simulink library "temp"  (Simulink 5.0)
undefined symbols (not defined in the file or in its folder): A, A1, B, B1, C, C1, D, D1, F, H, matrix, v1_vec, v2_vec, v3_vec, v_vec
libraries: aerolibschedule x46, simulink3 x46, simulink x18
(part 2 of 2)

== system temp/2D Controller Blend/K1 ==
  e = refs - y : Inport
  index_v1 : Inport  Port=2
  u_measured : Inport  Port=3
  v2 : Inport  Port=4
  Breakpoints v2 : simulink/Look-Up Tables/PreLook-Up Index Search  bpData=breakpoints_v2  searchMode=Binary Search  cacheBpFlag=on  outputFlag=off  extrapMode=Clip to Range  rangeErrorMode=None
  Controller indices1 : Subsystem
  Demux1 : Demux  Outputs=2
  K1 : Subsystem
  K2 : aerolibschedule/2D Controller Blend/K1/K1  SimViewingDevice=off  DataTypeOverride=UseLocalSettings  MinMaxOverflowLogging=UseLocalSettings
      settings: Permissions=ReadWrite  RTWFcnNameOpts=Auto  RTWFileNameOpts=Auto
  K3 : aerolibschedule/2D Controller Blend/K1/K1  SimViewingDevice=off  DataTypeOverride=UseLocalSettings  MinMaxOverflowLogging=UseLocalSettings
      settings: Permissions=ReadWrite  RTWFcnNameOpts=Auto  RTWFileNameOpts=Auto
  Sum1 : Sum  Inputs=+++  SaturateOnIntegerOverflow=on  InputSameDT=on
  lambda1 : Product  SaturateOnIntegerOverflow=on  InputSameDT=on
  lambda2 : Product  SaturateOnIntegerOverflow=on  InputSameDT=on
  lambda3 : Product  SaturateOnIntegerOverflow=on  InputSameDT=on
  u_demand : Outport
  wires:
  u_measured/1 -> K2/4, K3/4, K1/4(u_measured)
  e = refs - y/1 -> K2/1, K3/1, K1/1(e = refs - y)
  lambda2/1 -> Sum1/2
  lambda1/1 -> Sum1/1
  lambda3/1 -> Sum1/3
  K1/1(u_demand) -> lambda1/1
  K2/1 -> lambda2/1
  K3/1 -> lambda3/1
  Sum1/1 -> u_demand/1
  index_v1/1 -> K2/2, K3/2, K1/2(index1)
  Breakpoints v2/1 -> Demux1/1
  v2/1 -> Breakpoints v2/1
  Demux1/1 -> Controller indices1/1(index)
  Demux1/2 -> Controller indices1/2(lambda)
  Controller indices1/1(idx_K1) -> K1/3(index2)
  Controller indices1/2(lambda_K1) -> lambda1/2
  Controller indices1/3(idx_K2) -> K2/3
  Controller indices1/4(lambda_K2) -> lambda2/2
  Controller indices1/5(idx_K3) -> K3/3
  Controller indices1/6(lambda_K3) -> lambda3/2

== system temp/2D Observer Form [A(v),B(v),C(v),F(v),H(v)]/[A,B,C,F,H] ==
  y-y_dem : Inport
  AoA : Inport  Port=2  PortDimensions=2
  Mach : Inport  Port=3  PortDimensions=2
  u_meas : Inport  Port=4
  *A : Product  Multiplication=Matrix(*)  SaturateOnIntegerOverflow=on  InputSameDT=on
  *B : Product  Multiplication=Matrix(*)  SaturateOnIntegerOverflow=on  InputSameDT=on
  *C : Product  Multiplication=Matrix(*)  SaturateOnIntegerOverflow=on  InputSameDT=on
  *F : Product  Orientation=left  Multiplication=Matrix(*)  SaturateOnIntegerOverflow=on  InputSameDT=on
  *H : Product  Orientation=down  Multiplication=Matrix(*)  SaturateOnIntegerOverflow=on  InputSameDT=on
  A : aerolibschedule/Interpolate Matrix(x,y)  matrix=A
  B : aerolibschedule/Interpolate Matrix(x,y)  matrix=B
  C : aerolibschedule/Interpolate Matrix(x,y)  matrix=C
  F : aerolibschedule/Interpolate Matrix(x,y)  matrix=F
  H : aerolibschedule/Interpolate Matrix(x,y)  matrix=H
  Sum : Sum  Orientation=left  Inputs=+|+  SaturateOnIntegerOverflow=on  InputSameDT=on
  Sum1 : Sum  Orientation=down  Inputs=++|  SaturateOnIntegerOverflow=on  InputSameDT=on
  Sum2 : Sum  Orientation=down  Inputs=|++  SaturateOnIntegerOverflow=on  InputSameDT=on
  estimated state : Integrator  Orientation=left  InitialCondition=x_initial
  u_dem : Outport  Orientation=left
  wires:
  u_meas/1 -> *B/2
  Sum/1 -> estimated state/1
  estimated state/1 -> *F/2, *A/2, *C/2
  *A/1 -> Sum/2
  *F/1 -> u_dem/1
  *B/1 -> Sum1/1
  Sum1/1 -> Sum/1
  *H/1 -> Sum1/2
  Sum2/1 -> *H/2
  *C/1 -> Sum2/2
  A/1 -> *A/1
  C/1 -> *C/1
  F/1 -> *F/1
  B/1 -> *B/1
  H/1 -> *H/1
  y-y_dem/1 -> Sum2/1
  AoA/1 -> A/1, C/1, F/1, B/1, H/1
  Mach/1 -> A/2, C/2, F/2, B/2, H/2

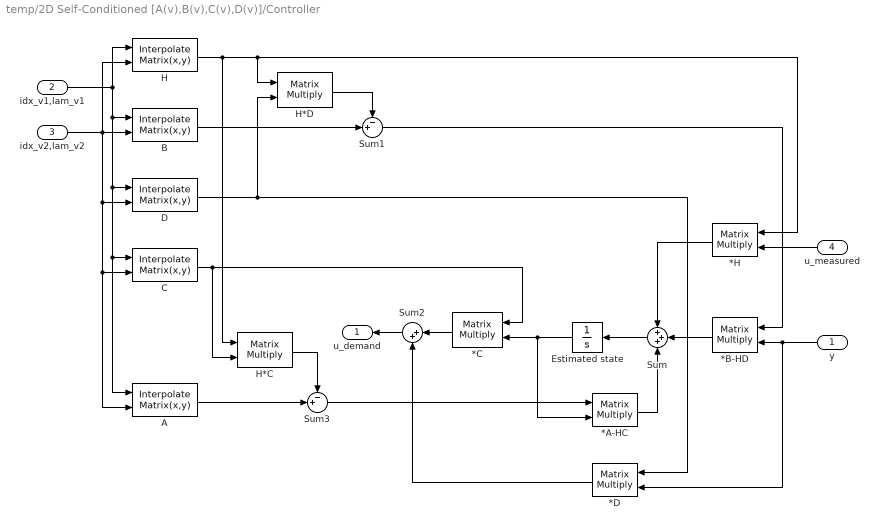
== system temp/2D Self-Conditioned [A(v),B(v),C(v),D(v)]/Controller ==
  y : Inport  Orientation=left
  idx_v1,lam_v1 : Inport  Port=2  PortDimensions=2
  idx_v2,lam_v2 : Inport  Port=3  PortDimensions=2
  u_measured : Inport  Orientation=left  Port=4
  *A-HC : Product  Multiplication=Matrix(*)  SaturateOnIntegerOverflow=on  InputSameDT=on
  *B-HD : Product  Orientation=left  Multiplication=Matrix(*)  SaturateOnIntegerOverflow=on  InputSameDT=on
  *C : Product  Orientation=left  Multiplication=Matrix(*)  SaturateOnIntegerOverflow=on  InputSameDT=on
  *D : Product  Orientation=left  Multiplication=Matrix(*)  SaturateOnIntegerOverflow=on  InputSameDT=on
  *H : Product  Orientation=left  Multiplication=Matrix(*)  SaturateOnIntegerOverflow=on  InputSameDT=on
  A : aerolibschedule/Interpolate Matrix(x,y)  matrix=A
  B : aerolibschedule/Interpolate Matrix(x,y)  matrix=B
  C : aerolibschedule/Interpolate Matrix(x,y)  matrix=C
  D : aerolibschedule/Interpolate Matrix(x,y)  matrix=D
  Estimated state : Integrator  Orientation=left  InitialCondition=x_initial
  H : aerolibschedule/Interpolate Matrix(x,y)  matrix=H
  H*C : Product  Multiplication=Matrix(*)  SaturateOnIntegerOverflow=on  InputSameDT=on
  H*D : Product  Multiplication=Matrix(*)  SaturateOnIntegerOverflow=on  InputSameDT=on
  Sum : Sum  Orientation=left  Inputs=+++  SaturateOnIntegerOverflow=on  InputSameDT=on
  Sum1 : Sum  Inputs=-+|  SaturateOnIntegerOverflow=on  InputSameDT=on
  Sum2 : Sum  Orientation=left  Inputs=|++  SaturateOnIntegerOverflow=on  InputSameDT=on
  Sum3 : Sum  Inputs=-+|  SaturateOnIntegerOverflow=on  InputSameDT=on
  u_demand : Outport  Orientation=left
  wires:
  idx_v2,lam_v2/1 -> C/2, A/2, D/2, H/2, B/2
  H*C/1 -> Sum3/1
  Sum3/1 -> *A-HC/1
  A/1 -> Sum3/2
  Sum1/1 -> *B-HD/1
  B/1 -> Sum1/2
  H*D/1 -> Sum1/1
  H/1 -> H*C/1, H*D/1, *H/1
  u_measured/1 -> *H/2
  *H/1 -> Sum/1
  *B-HD/1 -> Sum/2
  *A-HC/1 -> Sum/3
  Sum/1 -> Estimated state/1
  Estimated state/1 -> *C/2, *A-HC/2
  C/1 -> H*C/2, *C/1
  y/1 -> *B-HD/2, *D/2
  idx_v1,lam_v1/1 -> H/1, B/1, C/1, A/1, D/1
  *C/1 -> Sum2/1
  *D/1 -> Sum2/2
  Sum2/1 -> u_demand/1
  D/1 -> H*D/2, *D/1

== system temp/3D Controller [A(v),B(v),C(v),D(v)]/[A,B,C,D] ==
  y : Inport  Orientation=left
  AoA : Inport  Port=2  PortDimensions=2
  AoS : Inport  Port=3  PortDimensions=2
  Mach : Inport  Port=4  PortDimensions=2
  *A : Product  Multiplication=Matrix(*)  SaturateOnIntegerOverflow=on  InputSameDT=on
  *B : Product  Orientation=left  Multiplication=Matrix(*)  SaturateOnIntegerOverflow=on  InputSameDT=on
  *C : Product  Orientation=left  Multiplication=Matrix(*)  SaturateOnIntegerOverflow=on  InputSameDT=on
  *D : Product  Orientation=left  Multiplication=Matrix(*)  SaturateOnIntegerOverflow=on  InputSameDT=on
  A : aerolibschedule/Interpolate Matrix(x,y,z)  matrix=A
  B : aerolibschedule/Interpolate Matrix(x,y,z)  matrix=B
  C : aerolibschedule/Interpolate Matrix(x,y,z)  matrix=C
  D : aerolibschedule/Interpolate Matrix(x,y,z)  matrix=D
  Estimated state : Integrator  Orientation=left  InitialCondition=x_initial
  Sum : Sum  Orientation=left  Inputs=|++  SaturateOnIntegerOverflow=on  InputSameDT=on
  Sum2 : Sum  Orientation=left  Inputs=|++  SaturateOnIntegerOverflow=on  InputSameDT=on
  u : Outport  Orientation=left
  wires:
  D/1 -> *D/1
  Sum2/1 -> u/1
  *D/1 -> Sum2/2
  *C/1 -> Sum2/1
  Mach/1 -> C/3, A/3, D/3, B/3
  AoS/1 -> C/2, A/2, D/2, B/2
  AoA/1 -> C/1, A/1, D/1, B/1
  y/1 -> *D/2, *B/2
  B/1 -> *B/1
  C/1 -> *C/1
  A/1 -> *A/1
  *B/1 -> Sum/1
  *A/1 -> Sum/2
  Estimated state/1 -> *A/2, *C/2
  Sum/1 -> Estimated state/1

== system temp/3D Observer Form [A(v),B(v),C(v),F(v),H(v)]/[A,B,C,F,H] ==
  y-y_dem : Inport
  AoA : Inport  Port=2  PortDimensions=2
  AoS : Inport  Port=3  PortDimensions=2
  Mach : Inport  Port=4  PortDimensions=2
  u_meas : Inport  Port=5
  *A : Product  Multiplication=Matrix(*)  SaturateOnIntegerOverflow=on  InputSameDT=on
  *B : Product  Multiplication=Matrix(*)  SaturateOnIntegerOverflow=on  InputSameDT=on
  *C : Product  Multiplication=Matrix(*)  SaturateOnIntegerOverflow=on  InputSameDT=on
  *F : Product  Orientation=left  Multiplication=Matrix(*)  SaturateOnIntegerOverflow=on  InputSameDT=on
  *H : Product  Orientation=down  Multiplication=Matrix(*)  SaturateOnIntegerOverflow=on  InputSameDT=on
  A : aerolibschedule/Interpolate Matrix(x,y,z)  matrix=A
  B : aerolibschedule/Interpolate Matrix(x,y,z)  matrix=B
  C : aerolibschedule/Interpolate Matrix(x,y,z)  matrix=C
  F : aerolibschedule/Interpolate Matrix(x,y,z)  matrix=F
  H : aerolibschedule/Interpolate Matrix(x,y,z)  matrix=H
  Sum : Sum  Orientation=left  Inputs=+|+  SaturateOnIntegerOverflow=on  InputSameDT=on
  Sum1 : Sum  Orientation=down  Inputs=++|  SaturateOnIntegerOverflow=on  InputSameDT=on
  Sum2 : Sum  Orientation=down  Inputs=|++  SaturateOnIntegerOverflow=on  InputSameDT=on
  estimated state : Integrator  Orientation=left  InitialCondition=x_initial
  u_dem : Outport  Orientation=left
  wires:
  u_meas/1 -> *B/2
  Mach/1 -> A/3, C/3, F/3, B/3, H/3
  AoS/1 -> A/2, C/2, F/2, B/2, H/2
  AoA/1 -> A/1, C/1, F/1, B/1, H/1
  y-y_dem/1 -> Sum2/1
  H/1 -> *H/1
  B/1 -> *B/1
  F/1 -> *F/1
  C/1 -> *C/1
  A/1 -> *A/1
  *C/1 -> Sum2/2
  Sum2/1 -> *H/2
  *H/1 -> Sum1/2
  Sum1/1 -> Sum/1
  *B/1 -> Sum1/1
  *F/1 -> u_dem/1
  *A/1 -> Sum/2
  estimated state/1 -> *C/2, *A/2, *F/2
  Sum/1 -> estimated state/1

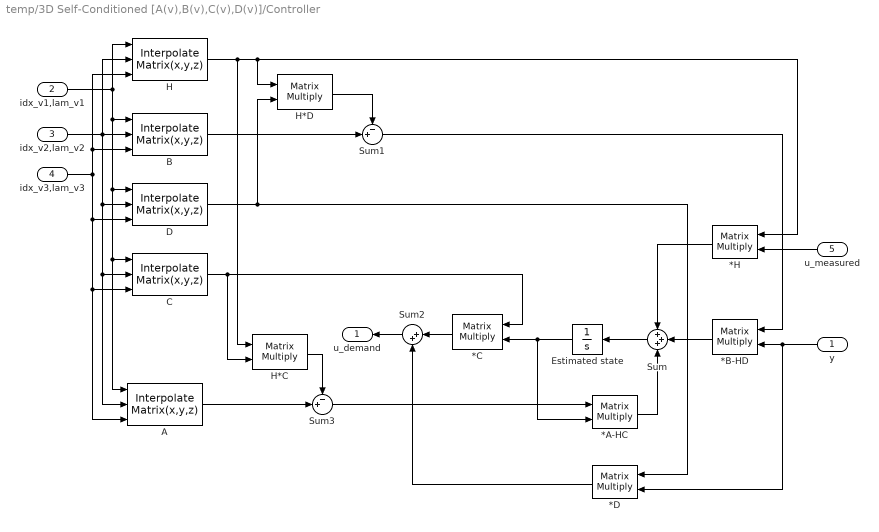
== system temp/3D Self-Conditioned [A(v),B(v),C(v),D(v)]/Controller ==
  y : Inport  Orientation=left
  idx_v1,lam_v1 : Inport  Port=2  PortDimensions=2
  idx_v2,lam_v2 : Inport  Port=3  PortDimensions=2
  idx_v3,lam_v3 : Inport  Port=4  PortDimensions=2
  u_measured : Inport  Orientation=left  Port=5
  *A-HC : Product  Multiplication=Matrix(*)  SaturateOnIntegerOverflow=on  InputSameDT=on
  *B-HD : Product  Orientation=left  Multiplication=Matrix(*)  SaturateOnIntegerOverflow=on  InputSameDT=on
  *C : Product  Orientation=left  Multiplication=Matrix(*)  SaturateOnIntegerOverflow=on  InputSameDT=on
  *D : Product  Orientation=left  Multiplication=Matrix(*)  SaturateOnIntegerOverflow=on  InputSameDT=on
  *H : Product  Orientation=left  Multiplication=Matrix(*)  SaturateOnIntegerOverflow=on  InputSameDT=on
  A : aerolibschedule/Interpolate Matrix(x,y,z)  matrix=A
  B : aerolibschedule/Interpolate Matrix(x,y,z)  matrix=B
  C : aerolibschedule/Interpolate Matrix(x,y,z)  matrix=C
  D : aerolibschedule/Interpolate Matrix(x,y,z)  matrix=D
  Estimated state : Integrator  Orientation=left  InitialCondition=x_initial
  H : aerolibschedule/Interpolate Matrix(x,y,z)  matrix=H
  H*C : Product  Multiplication=Matrix(*)  SaturateOnIntegerOverflow=on  InputSameDT=on
  H*D : Product  Multiplication=Matrix(*)  SaturateOnIntegerOverflow=on  InputSameDT=on
  Sum : Sum  Orientation=left  Inputs=+++  SaturateOnIntegerOverflow=on  InputSameDT=on
  Sum1 : Sum  Inputs=-+|  SaturateOnIntegerOverflow=on  InputSameDT=on
  Sum2 : Sum  Orientation=left  Inputs=|++  SaturateOnIntegerOverflow=on  InputSameDT=on
  Sum3 : Sum  Inputs=-+|  SaturateOnIntegerOverflow=on  InputSameDT=on
  u_demand : Outport  Orientation=left
  wires:
  idx_v3,lam_v3/1 -> C/3, A/3, D/3, H/3, B/3
  D/1 -> *D/1, H*D/2
  Sum2/1 -> u_demand/1
  *D/1 -> Sum2/2
  *C/1 -> Sum2/1
  idx_v1,lam_v1/1 -> C/1, A/1, D/1, H/1, B/1
  y/1 -> *D/2, *B-HD/2
  C/1 -> *C/1, H*C/2
  Estimated state/1 -> *A-HC/2, *C/2
  Sum/1 -> Estimated state/1
  *A-HC/1 -> Sum/3
  *B-HD/1 -> Sum/2
  *H/1 -> Sum/1
  u_measured/1 -> *H/2
  H/1 -> *H/1, H*D/1, H*C/1
  H*D/1 -> Sum1/1
  B/1 -> Sum1/2
  Sum1/1 -> *B-HD/1
  A/1 -> Sum3/2
  Sum3/1 -> *A-HC/1
  H*C/1 -> Sum3/1
  idx_v2,lam_v2/1 -> C/2, A/2, D/2, H/2, B/2

== system temp/Interpolate Matrix(x)/Matrix interpolation ==
  index : Inport
  lambda_x : Inport  Orientation=down  Port=2  PortDimensions=1
  1-lambda_x : Product  SaturateOnIntegerOverflow=on  InputSameDT=on
  Fcn : Fcn  Expr=1-u(1)
  Sum : Sum  Inputs=|++  SaturateOnIntegerOverflow=on  InputSameDT=on
  Sum3 : Sum  Inputs=+|+  SaturateOnIntegerOverflow=on  InputSameDT=on
  "[0]" : simulink3/Functions & Tables/Direct Look-Up Table (n-D)  maskTabDims=More...  explicitNumDims=3  outDims=2-D Matrix  tabIsInput=off  mxTable=matrix  clipFlag=Warning
  "[1]" : simulink3/Functions & Tables/Direct Look-Up Table (n-D)  maskTabDims=More...  explicitNumDims=3  outDims=2-D Matrix  tabIsInput=off  mxTable=matrix  clipFlag=Warning
  lambda_x. : Product  SaturateOnIntegerOverflow=on  InputSameDT=on
  offset for upper index 1 : Constant
  matrix : Outport
  wires:
  Sum3/1 -> matrix/1
  lambda_x./1 -> Sum3/2
  1-lambda_x/1 -> Sum3/1
  Fcn/1 -> 1-lambda_x/2
  "[1]"/1 -> lambda_x./1
  "[0]"/1 -> 1-lambda_x/1
  Sum/1 -> "[1]"/1
  offset for upper index 1/1 -> Sum/2
  index/1 -> "[0]"/1, Sum/1
  lambda_x/1 -> lambda_x./2, Fcn/1

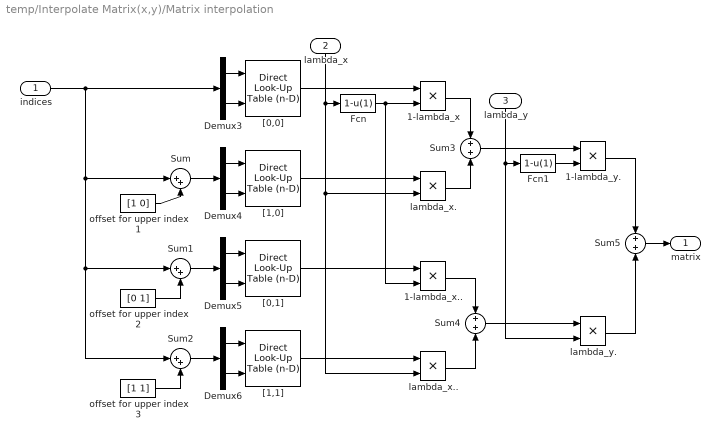
== system temp/Interpolate Matrix(x,y)/Matrix interpolation ==
  indices : Inport
  lambda_x : Inport  Orientation=down  Port=2
  lambda_y : Inport  Orientation=down  Port=3
  1-lambda_x : Product  SaturateOnIntegerOverflow=on  InputSameDT=on
  1-lambda_x.. : Product  SaturateOnIntegerOverflow=on  InputSameDT=on
  1-lambda_y. : Product  SaturateOnIntegerOverflow=on  InputSameDT=on
  Demux{3..6} (4 alike) : Demux  Outputs=2
  Fcn : Fcn  Expr=1-u(1)
  Fcn1 : Fcn  Expr=1-u(1)
  Sum : Sum  Inputs=|++  SaturateOnIntegerOverflow=on  InputSameDT=on
  Sum1 : Sum  Inputs=|++  SaturateOnIntegerOverflow=on  InputSameDT=on
  Sum2 : Sum  Inputs=|++  SaturateOnIntegerOverflow=on  InputSameDT=on
  Sum3 : Sum  Inputs=+|+  SaturateOnIntegerOverflow=on  InputSameDT=on
  Sum4 : Sum  Inputs=+|+  SaturateOnIntegerOverflow=on  InputSameDT=on
  Sum5 : Sum  Inputs=+|+  SaturateOnIntegerOverflow=on  InputSameDT=on
  "[0,0]" : simulink3/Functions & Tables/Direct Look-Up Table (n-D)  maskTabDims=More...  explicitNumDims=4  outDims=2-D Matrix  tabIsInput=off  mxTable=matrix  clipFlag=Warning
  "[0,1]" : simulink3/Functions & Tables/Direct Look-Up Table (n-D)  maskTabDims=More...  explicitNumDims=4  outDims=2-D Matrix  tabIsInput=off  mxTable=matrix  clipFlag=Warning
  "[1,0]" : simulink3/Functions & Tables/Direct Look-Up Table (n-D)  maskTabDims=More...  explicitNumDims=4  outDims=2-D Matrix  tabIsInput=off  mxTable=matrix  clipFlag=Warning
  "[1,1]" : simulink3/Functions & Tables/Direct Look-Up Table (n-D)  maskTabDims=More...  explicitNumDims=4  outDims=2-D Matrix  tabIsInput=off  mxTable=matrix  clipFlag=Warning
  lambda_x. : Product  SaturateOnIntegerOverflow=on  InputSameDT=on
  lambda_x.. : Product  SaturateOnIntegerOverflow=on  InputSameDT=on
  lambda_y. : Product  SaturateOnIntegerOverflow=on  InputSameDT=on
  offset for upper index 1 : Constant  Value=[1 0]
  offset for upper index 2 : Constant  Value=[0 1]
  offset for upper index 3 : Constant  Value=[1 1]
  matrix : Outport
  wires:
  lambda_x/1 -> lambda_x../2, lambda_x./2, Fcn/1
  lambda_y/1 -> lambda_y./2, Fcn1/1
  Sum5/1 -> matrix/1
  indices/1 -> Sum2/1, Sum1/1, Sum/1, Demux3/1
  offset for upper index 3/1 -> Sum2/2
  Sum2/1 -> Demux6/1
  Demux6/2 -> "[1,1]"/2
  Demux6/1 -> "[1,1]"/1
  offset for upper index 2/1 -> Sum1/2
  Sum1/1 -> Demux5/1
  Demux5/2 -> "[0,1]"/2
  Demux5/1 -> "[0,1]"/1
  offset for upper index 1/1 -> Sum/2
  Sum/1 -> Demux4/1
  Demux4/2 -> "[1,0]"/2
  Demux4/1 -> "[1,0]"/1
  Demux3/2 -> "[0,0]"/2
  Demux3/1 -> "[0,0]"/1
  "[0,0]"/1 -> 1-lambda_x/1
  "[1,0]"/1 -> lambda_x./1
  "[0,1]"/1 -> 1-lambda_x../1
  "[1,1]"/1 -> lambda_x../1
  Fcn/1 -> 1-lambda_x/2, 1-lambda_x../2
  1-lambda_x/1 -> Sum3/1
  lambda_x./1 -> Sum3/2
  1-lambda_x../1 -> Sum4/1
  lambda_x../1 -> Sum4/2
  Sum3/1 -> 1-lambda_y./1
  Sum4/1 -> lambda_y./1
  Fcn1/1 -> 1-lambda_y./2
  1-lambda_y./1 -> Sum5/1
  lambda_y./1 -> Sum5/2

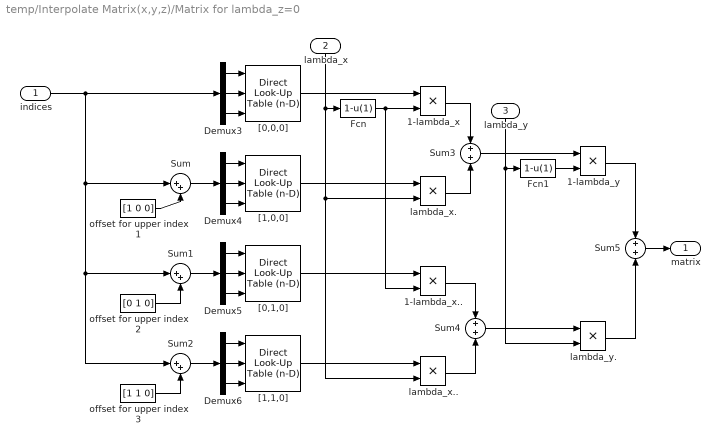
== system temp/Interpolate Matrix(x,y,z)/Matrix for lambda_z=0 ==
  indices : Inport
  lambda_x : Inport  Orientation=down  Port=2
  lambda_y : Inport  Orientation=down  Port=3
  1-lambda_x : Product  SaturateOnIntegerOverflow=on  InputSameDT=on
  1-lambda_x.. : Product  SaturateOnIntegerOverflow=on  InputSameDT=on
  1-lambda_y : Product  SaturateOnIntegerOverflow=on  InputSameDT=on
  Demux{3..6} (4 alike) : Demux  Outputs=3
  Fcn : Fcn  Expr=1-u(1)
  Fcn1 : Fcn  Expr=1-u(1)
  Sum : Sum  Inputs=|++  SaturateOnIntegerOverflow=on  InputSameDT=on
  Sum1 : Sum  Inputs=|++  SaturateOnIntegerOverflow=on  InputSameDT=on
  Sum2 : Sum  Inputs=|++  SaturateOnIntegerOverflow=on  InputSameDT=on
  Sum3 : Sum  Inputs=+|+  SaturateOnIntegerOverflow=on  InputSameDT=on
  Sum4 : Sum  Inputs=+|+  SaturateOnIntegerOverflow=on  InputSameDT=on
  Sum5 : Sum  Inputs=+|+  SaturateOnIntegerOverflow=on  InputSameDT=on
  "[0,0,0]" : simulink3/Functions & Tables/Direct Look-Up Table (n-D)  maskTabDims=More...  explicitNumDims=5  outDims=2-D Matrix  tabIsInput=off  mxTable=matrix  clipFlag=Warning
  "[0,1,0]" : simulink3/Functions & Tables/Direct Look-Up Table (n-D)  maskTabDims=More...  explicitNumDims=5  outDims=2-D Matrix  tabIsInput=off  mxTable=matrix  clipFlag=Warning
  "[1,0,0]" : simulink3/Functions & Tables/Direct Look-Up Table (n-D)  maskTabDims=More...  explicitNumDims=5  outDims=2-D Matrix  tabIsInput=off  mxTable=matrix  clipFlag=Warning
  "[1,1,0]" : simulink3/Functions & Tables/Direct Look-Up Table (n-D)  maskTabDims=More...  explicitNumDims=5  outDims=2-D Matrix  tabIsInput=off  mxTable=matrix  clipFlag=Warning
  lambda_x. : Product  SaturateOnIntegerOverflow=on  InputSameDT=on
  lambda_x.. : Product  SaturateOnIntegerOverflow=on  InputSameDT=on
  lambda_y. : Product  SaturateOnIntegerOverflow=on  InputSameDT=on
  offset for upper index 1 : Constant  Value=[1 0 0]
  offset for upper index 2 : Constant  Value=[0 1 0]
  offset for upper index 3 : Constant  Value=[1 1 0]
  matrix : Outport
  wires:
  lambda_x/1 -> lambda_x../2, lambda_x./2, Fcn/1
  lambda_y/1 -> lambda_y./2, Fcn1/1
  lambda_y./1 -> Sum5/2
  1-lambda_y/1 -> Sum5/1
  Fcn1/1 -> 1-lambda_y/2
  Sum4/1 -> lambda_y./1
  Sum3/1 -> 1-lambda_y/1
  lambda_x../1 -> Sum4/2
  1-lambda_x../1 -> Sum4/1
  lambda_x./1 -> Sum3/2
  1-lambda_x/1 -> Sum3/1
  Fcn/1 -> 1-lambda_x../2, 1-lambda_x/2
  "[1,1,0]"/1 -> lambda_x../1
  "[0,1,0]"/1 -> 1-lambda_x../1
  "[1,0,0]"/1 -> lambda_x./1
  "[0,0,0]"/1 -> 1-lambda_x/1
  Demux3/1 -> "[0,0,0]"/1
  Demux3/2 -> "[0,0,0]"/2
  Demux3/3 -> "[0,0,0]"/3
  Demux4/1 -> "[1,0,0]"/1
  Demux4/2 -> "[1,0,0]"/2
  Sum/1 -> Demux4/1
  Demux4/3 -> "[1,0,0]"/3
  offset for upper index 1/1 -> Sum/2
  Demux5/1 -> "[0,1,0]"/1
  Demux5/2 -> "[0,1,0]"/2
  Demux5/3 -> "[0,1,0]"/3
  Sum1/1 -> Demux5/1
  offset for upper index 2/1 -> Sum1/2
  Demux6/1 -> "[1,1,0]"/1
  Demux6/2 -> "[1,1,0]"/2
  Demux6/3 -> "[1,1,0]"/3
  Sum2/1 -> Demux6/1
  offset for upper index 3/1 -> Sum2/2
  indices/1 -> Demux3/1, Sum/1, Sum1/1, Sum2/1
  Sum5/1 -> matrix/1

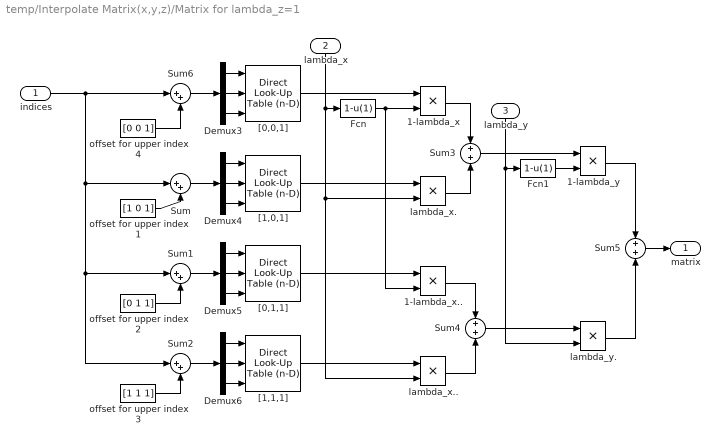
== system temp/Interpolate Matrix(x,y,z)/Matrix for lambda_z=1 ==
  indices : Inport
  lambda_x : Inport  Orientation=down  Port=2
  lambda_y : Inport  Orientation=down  Port=3
  1-lambda_x : Product  SaturateOnIntegerOverflow=on  InputSameDT=on
  1-lambda_x.. : Product  SaturateOnIntegerOverflow=on  InputSameDT=on
  1-lambda_y : Product  SaturateOnIntegerOverflow=on  InputSameDT=on
  Demux{3..6} (4 alike) : Demux  Outputs=3
  Fcn : Fcn  Expr=1-u(1)
  Fcn1 : Fcn  Expr=1-u(1)
  Sum{,1..2,6} (4 alike) : Sum  Inputs=|++  SaturateOnIntegerOverflow=on  InputSameDT=on
  Sum3 : Sum  Inputs=+|+  SaturateOnIntegerOverflow=on  InputSameDT=on
  Sum4 : Sum  Inputs=+|+  SaturateOnIntegerOverflow=on  InputSameDT=on
  Sum5 : Sum  Inputs=+|+  SaturateOnIntegerOverflow=on  InputSameDT=on
  "[0,0,1]" : simulink3/Functions & Tables/Direct Look-Up Table (n-D)  maskTabDims=More...  explicitNumDims=5  outDims=2-D Matrix  tabIsInput=off  mxTable=matrix  clipFlag=Warning
  "[0,1,1]" : simulink3/Functions & Tables/Direct Look-Up Table (n-D)  maskTabDims=More...  explicitNumDims=5  outDims=2-D Matrix  tabIsInput=off  mxTable=matrix  clipFlag=Warning
  "[1,0,1]" : simulink3/Functions & Tables/Direct Look-Up Table (n-D)  maskTabDims=More...  explicitNumDims=5  outDims=2-D Matrix  tabIsInput=off  mxTable=matrix  clipFlag=Warning
  "[1,1,1]" : simulink3/Functions & Tables/Direct Look-Up Table (n-D)  maskTabDims=More...  explicitNumDims=5  outDims=2-D Matrix  tabIsInput=off  mxTable=matrix  clipFlag=Warning
  lambda_x. : Product  SaturateOnIntegerOverflow=on  InputSameDT=on
  lambda_x.. : Product  SaturateOnIntegerOverflow=on  InputSameDT=on
  lambda_y. : Product  SaturateOnIntegerOverflow=on  InputSameDT=on
  offset for upper index 1 : Constant  Value=[1 0 1]
  offset for upper index 2 : Constant  Value=[0 1 1]
  offset for upper index 3 : Constant  Value=[1 1 1]
  offset for upper index 4 : Constant  Value=[0 0 1]
  matrix : Outport
  wires:
  offset for upper index 4/1 -> Sum6/2
  Sum6/1 -> Demux3/1
  Sum5/1 -> matrix/1
  indices/1 -> Sum6/1, Sum2/1, Sum1/1, Sum/1
  offset for upper index 3/1 -> Sum2/2
  Sum2/1 -> Demux6/1
  Demux6/3 -> "[1,1,1]"/3
  Demux6/2 -> "[1,1,1]"/2
  Demux6/1 -> "[1,1,1]"/1
  offset for upper index 2/1 -> Sum1/2
  Sum1/1 -> Demux5/1
  Demux5/3 -> "[0,1,1]"/3
  Demux5/2 -> "[0,1,1]"/2
  Demux5/1 -> "[0,1,1]"/1
  offset for upper index 1/1 -> Sum/2
  Demux4/3 -> "[1,0,1]"/3
  Sum/1 -> Demux4/1
  Demux4/2 -> "[1,0,1]"/2
  Demux4/1 -> "[1,0,1]"/1
  Demux3/3 -> "[0,0,1]"/3
  Demux3/2 -> "[0,0,1]"/2
  Demux3/1 -> "[0,0,1]"/1
  "[0,0,1]"/1 -> 1-lambda_x/1
  "[1,0,1]"/1 -> lambda_x./1
  "[0,1,1]"/1 -> 1-lambda_x../1
  "[1,1,1]"/1 -> lambda_x../1
  Fcn/1 -> 1-lambda_x/2, 1-lambda_x../2
  1-lambda_x/1 -> Sum3/1
  lambda_x./1 -> Sum3/2
  1-lambda_x../1 -> Sum4/1
  lambda_x../1 -> Sum4/2
  Sum3/1 -> 1-lambda_y/1
  Sum4/1 -> lambda_y./1
  Fcn1/1 -> 1-lambda_y/2
  1-lambda_y/1 -> Sum5/1
  lambda_y./1 -> Sum5/2
  lambda_y/1 -> Fcn1/1, lambda_y./2
  lambda_x/1 -> Fcn/1, lambda_x./2, lambda_x../2

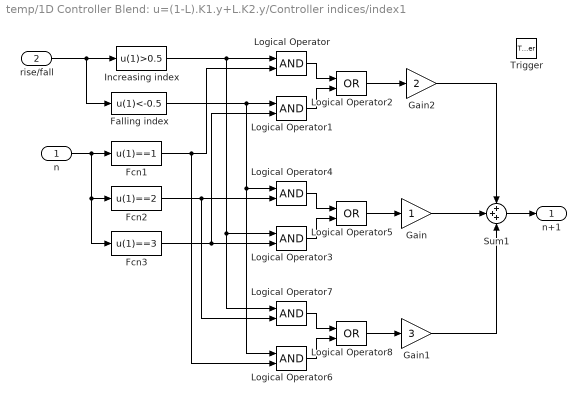
== system temp/1D Controller Blend: u=(1-L).K1.y+L.K2.y/Controller indices/index1 ==
  n : Inport
  rise/fall : Inport  Port=2
  Trigger : TriggerPort
  Falling index : Fcn  Expr=u(1)<-0.5
  Fcn1 : Fcn  Expr=u(1)==1
  Fcn2 : Fcn  Expr=u(1)==2
  Fcn3 : Fcn  Expr=u(1)==3
  Gain : Gain  SaturateOnIntegerOverflow=on
  Gain1 : Gain  Gain=3  SaturateOnIntegerOverflow=on
  Gain2 : Gain  Gain=2  SaturateOnIntegerOverflow=on
  Increasing index : Fcn  Expr=u(1)>0.5
  Logical Operator{,1,3..4,6..7} (6 alike) : Logic  ShowAdditionalParam=on  AllPortsSameDT=off
  Logical Operator2 : Logic  Operator=OR  ShowAdditionalParam=on  AllPortsSameDT=off  OutDataTypeMode=Specify via dialog  LogicDataType=float('double')
  Logical Operator5 : Logic  Operator=OR  ShowAdditionalParam=on  AllPortsSameDT=off  OutDataTypeMode=Specify via dialog  LogicDataType=float('double')
  Logical Operator8 : Logic  Operator=OR  ShowAdditionalParam=on  AllPortsSameDT=off  OutDataTypeMode=Specify via dialog  LogicDataType=float('double')
  Sum1 : Sum  Inputs=+++  SaturateOnIntegerOverflow=on  InputSameDT=on
  n+1 : Outport  InitialOutput=1
  wires:
  rise/fall/1 -> Falling index/1, Increasing index/1
  Gain2/1 -> Sum1/1
  Gain1/1 -> Sum1/3
  Logical Operator8/1 -> Gain1/1
  Logical Operator6/1 -> Logical Operator8/2
  Logical Operator7/1 -> Logical Operator8/1
  Gain/1 -> Sum1/2
  Logical Operator5/1 -> Gain/1
  Logical Operator3/1 -> Logical Operator5/2
  Logical Operator4/1 -> Logical Operator5/1
  Fcn2/1 -> Logical Operator7/2, Logical Operator4/2
  Logical Operator2/1 -> Gain2/1
  Sum1/1 -> n+1/1
  Logical Operator1/1 -> Logical Operator2/2
  Logical Operator/1 -> Logical Operator2/1
  Fcn3/1 -> Logical Operator3/2, Logical Operator1/2
  Falling index/1 -> Logical Operator6/1, Logical Operator4/1, Logical Operator1/1
  Fcn1/1 -> Logical Operator6/2, Logical Operator/2
  Increasing index/1 -> Logical Operator7/1, Logical Operator3/1, Logical Operator/1
  n/1 -> Fcn1/1, Fcn3/1, Fcn2/1

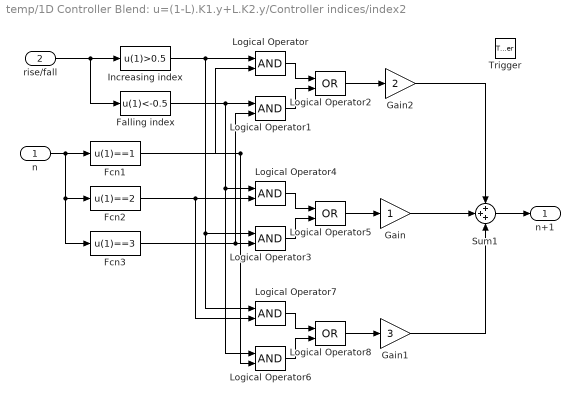
== system temp/1D Controller Blend: u=(1-L).K1.y+L.K2.y/Controller indices/index2 ==
  n : Inport
  rise/fall : Inport  Port=2
  Trigger : TriggerPort
  Falling index : Fcn  Expr=u(1)<-0.5
  Fcn1 : Fcn  Expr=u(1)==1
  Fcn2 : Fcn  Expr=u(1)==2
  Fcn3 : Fcn  Expr=u(1)==3
  Gain : Gain  SaturateOnIntegerOverflow=on
  Gain1 : Gain  Gain=3  SaturateOnIntegerOverflow=on
  Gain2 : Gain  Gain=2  SaturateOnIntegerOverflow=on
  Increasing index : Fcn  Expr=u(1)>0.5
  Logical Operator{,1,3..4,6..7} (6 alike) : Logic  ShowAdditionalParam=on  AllPortsSameDT=off
  Logical Operator2 : Logic  Operator=OR  ShowAdditionalParam=on  AllPortsSameDT=off  OutDataTypeMode=Specify via dialog  LogicDataType=float('double')
  Logical Operator5 : Logic  Operator=OR  ShowAdditionalParam=on  AllPortsSameDT=off  OutDataTypeMode=Specify via dialog  LogicDataType=float('double')
  Logical Operator8 : Logic  Operator=OR  ShowAdditionalParam=on  AllPortsSameDT=off  OutDataTypeMode=Specify via dialog  LogicDataType=float('double')
  Sum1 : Sum  Inputs=+++  SaturateOnIntegerOverflow=on  InputSameDT=on
  n+1 : Outport  InitialOutput=2
  wires:
  n/1 -> Fcn1/1, Fcn2/1, Fcn3/1
  Increasing index/1 -> Logical Operator/1, Logical Operator3/1, Logical Operator7/1
  Fcn1/1 -> Logical Operator/2, Logical Operator6/2
  Falling index/1 -> Logical Operator1/1, Logical Operator4/1, Logical Operator6/1
  Fcn3/1 -> Logical Operator1/2, Logical Operator3/2
  Logical Operator/1 -> Logical Operator2/1
  Logical Operator1/1 -> Logical Operator2/2
  Sum1/1 -> n+1/1
  Logical Operator2/1 -> Gain2/1
  Fcn2/1 -> Logical Operator4/2, Logical Operator7/2
  Logical Operator4/1 -> Logical Operator5/1
  Logical Operator3/1 -> Logical Operator5/2
  Logical Operator5/1 -> Gain/1
  Gain/1 -> Sum1/2
  Logical Operator7/1 -> Logical Operator8/1
  Logical Operator6/1 -> Logical Operator8/2
  Logical Operator8/1 -> Gain1/1
  Gain1/1 -> Sum1/3
  Gain2/1 -> Sum1/1
  rise/fall/1 -> Increasing index/1, Falling index/1

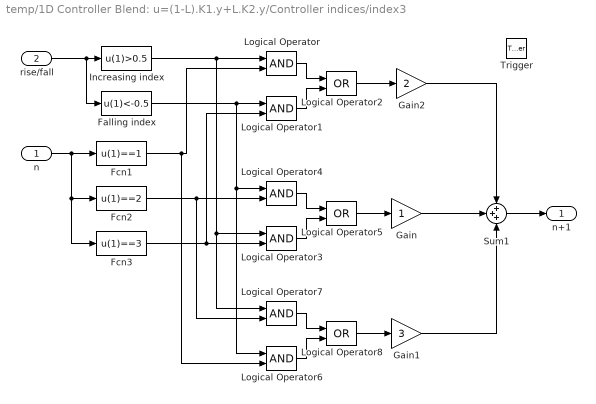
== system temp/1D Controller Blend: u=(1-L).K1.y+L.K2.y/Controller indices/index3 ==
  n : Inport
  rise/fall : Inport  Port=2
  Trigger : TriggerPort
  Falling index : Fcn  Expr=u(1)<-0.5
  Fcn1 : Fcn  Expr=u(1)==1
  Fcn2 : Fcn  Expr=u(1)==2
  Fcn3 : Fcn  Expr=u(1)==3
  Gain : Gain  SaturateOnIntegerOverflow=on
  Gain1 : Gain  Gain=3  SaturateOnIntegerOverflow=on
  Gain2 : Gain  Gain=2  SaturateOnIntegerOverflow=on
  Increasing index : Fcn  Expr=u(1)>0.5
  Logical Operator{,1,3..4,6..7} (6 alike) : Logic  ShowAdditionalParam=on  AllPortsSameDT=off
  Logical Operator2 : Logic  Operator=OR  ShowAdditionalParam=on  AllPortsSameDT=off  OutDataTypeMode=Specify via dialog  LogicDataType=float('double')
  Logical Operator5 : Logic  Operator=OR  ShowAdditionalParam=on  AllPortsSameDT=off  OutDataTypeMode=Specify via dialog  LogicDataType=float('double')
  Logical Operator8 : Logic  Operator=OR  ShowAdditionalParam=on  AllPortsSameDT=off  OutDataTypeMode=Specify via dialog  LogicDataType=float('double')
  Sum1 : Sum  Inputs=+++  SaturateOnIntegerOverflow=on  InputSameDT=on
  n+1 : Outport  InitialOutput=3
  wires:
  rise/fall/1 -> Falling index/1, Increasing index/1
  Gain2/1 -> Sum1/1
  Gain1/1 -> Sum1/3
  Logical Operator8/1 -> Gain1/1
  Logical Operator6/1 -> Logical Operator8/2
  Logical Operator7/1 -> Logical Operator8/1
  Gain/1 -> Sum1/2
  Logical Operator5/1 -> Gain/1
  Logical Operator3/1 -> Logical Operator5/2
  Logical Operator4/1 -> Logical Operator5/1
  Fcn2/1 -> Logical Operator7/2, Logical Operator4/2
  Logical Operator2/1 -> Gain2/1
  Sum1/1 -> n+1/1
  Logical Operator1/1 -> Logical Operator2/2
  Logical Operator/1 -> Logical Operator2/1
  Fcn3/1 -> Logical Operator3/2, Logical Operator1/2
  Falling index/1 -> Logical Operator6/1, Logical Operator4/1, Logical Operator1/1
  Fcn1/1 -> Logical Operator6/2, Logical Operator/2
  Increasing index/1 -> Logical Operator7/1, Logical Operator3/1, Logical Operator/1
  n/1 -> Fcn1/1, Fcn2/1, Fcn3/1

== system temp/2D Controller Blend/Controller indices1/index1 ==
  n : Inport
  rise/fall : Inport  Port=2
  Trigger : TriggerPort
  Falling index : Fcn  Expr=u(1)<-0.5
  Fcn1 : Fcn  Expr=u(1)==1
  Fcn2 : Fcn  Expr=u(1)==2
  Fcn3 : Fcn  Expr=u(1)==3
  Gain : Gain  SaturateOnIntegerOverflow=on
  Gain1 : Gain  Gain=3  SaturateOnIntegerOverflow=on
  Gain2 : Gain  Gain=2  SaturateOnIntegerOverflow=on
  Increasing index : Fcn  Expr=u(1)>0.5
  Logical Operator{,1,3..4,6..7} (6 alike) : Logic  ShowAdditionalParam=on  AllPortsSameDT=off
  Logical Operator2 : Logic  Operator=OR  ShowAdditionalParam=on  AllPortsSameDT=off  OutDataTypeMode=Specify via dialog  LogicDataType=float('double')
  Logical Operator5 : Logic  Operator=OR  ShowAdditionalParam=on  AllPortsSameDT=off  OutDataTypeMode=Specify via dialog  LogicDataType=float('double')
  Logical Operator8 : Logic  Operator=OR  ShowAdditionalParam=on  AllPortsSameDT=off  OutDataTypeMode=Specify via dialog  LogicDataType=float('double')
  Sum1 : Sum  Inputs=+++  SaturateOnIntegerOverflow=on  InputSameDT=on
  n+1 : Outport  InitialOutput=1
  wires:
  rise/fall/1 -> Falling index/1, Increasing index/1
  Gain2/1 -> Sum1/1
  Gain1/1 -> Sum1/3
  Logical Operator8/1 -> Gain1/1
  Logical Operator6/1 -> Logical Operator8/2
  Logical Operator7/1 -> Logical Operator8/1
  Gain/1 -> Sum1/2
  Logical Operator5/1 -> Gain/1
  Logical Operator3/1 -> Logical Operator5/2
  Logical Operator4/1 -> Logical Operator5/1
  Fcn2/1 -> Logical Operator7/2, Logical Operator4/2
  Logical Operator2/1 -> Gain2/1
  Sum1/1 -> n+1/1
  Logical Operator1/1 -> Logical Operator2/2
  Logical Operator/1 -> Logical Operator2/1
  Fcn3/1 -> Logical Operator3/2, Logical Operator1/2
  Falling index/1 -> Logical Operator6/1, Logical Operator4/1, Logical Operator1/1
  Fcn1/1 -> Logical Operator6/2, Logical Operator/2
  Increasing index/1 -> Logical Operator7/1, Logical Operator3/1, Logical Operator/1
  n/1 -> Fcn3/1, Fcn2/1, Fcn1/1

== system temp/2D Controller Blend/Controller indices1/index2 ==
  n : Inport
  rise/fall : Inport  Port=2
  Trigger : TriggerPort
  Falling index : Fcn  Expr=u(1)<-0.5
  Fcn1 : Fcn  Expr=u(1)==1
  Fcn2 : Fcn  Expr=u(1)==2
  Fcn3 : Fcn  Expr=u(1)==3
  Gain : Gain  SaturateOnIntegerOverflow=on
  Gain1 : Gain  Gain=3  SaturateOnIntegerOverflow=on
  Gain2 : Gain  Gain=2  SaturateOnIntegerOverflow=on
  Increasing index : Fcn  Expr=u(1)>0.5
  Logical Operator{,1,3..4,6..7} (6 alike) : Logic  ShowAdditionalParam=on  AllPortsSameDT=off
  Logical Operator2 : Logic  Operator=OR  ShowAdditionalParam=on  AllPortsSameDT=off  OutDataTypeMode=Specify via dialog  LogicDataType=float('double')
  Logical Operator5 : Logic  Operator=OR  ShowAdditionalParam=on  AllPortsSameDT=off  OutDataTypeMode=Specify via dialog  LogicDataType=float('double')
  Logical Operator8 : Logic  Operator=OR  ShowAdditionalParam=on  AllPortsSameDT=off  OutDataTypeMode=Specify via dialog  LogicDataType=float('double')
  Sum1 : Sum  Inputs=+++  SaturateOnIntegerOverflow=on  InputSameDT=on
  n+1 : Outport  InitialOutput=2
  wires:
  n/1 -> Fcn1/1, Fcn2/1, Fcn3/1
  Increasing index/1 -> Logical Operator/1, Logical Operator3/1, Logical Operator7/1
  Fcn1/1 -> Logical Operator/2, Logical Operator6/2
  Falling index/1 -> Logical Operator1/1, Logical Operator4/1, Logical Operator6/1
  Fcn3/1 -> Logical Operator1/2, Logical Operator3/2
  Logical Operator/1 -> Logical Operator2/1
  Logical Operator1/1 -> Logical Operator2/2
  Sum1/1 -> n+1/1
  Logical Operator2/1 -> Gain2/1
  Fcn2/1 -> Logical Operator4/2, Logical Operator7/2
  Logical Operator4/1 -> Logical Operator5/1
  Logical Operator3/1 -> Logical Operator5/2
  Logical Operator5/1 -> Gain/1
  Gain/1 -> Sum1/2
  Logical Operator7/1 -> Logical Operator8/1
  Logical Operator6/1 -> Logical Operator8/2
  Logical Operator8/1 -> Gain1/1
  Gain1/1 -> Sum1/3
  Gain2/1 -> Sum1/1
  rise/fall/1 -> Increasing index/1, Falling index/1

== system temp/2D Controller Blend/Controller indices1/index3 ==
  n : Inport
  rise/fall : Inport  Port=2
  Trigger : TriggerPort
  Falling index : Fcn  Expr=u(1)<-0.5
  Fcn1 : Fcn  Expr=u(1)==1
  Fcn2 : Fcn  Expr=u(1)==2
  Fcn3 : Fcn  Expr=u(1)==3
  Gain : Gain  SaturateOnIntegerOverflow=on
  Gain1 : Gain  Gain=3  SaturateOnIntegerOverflow=on
  Gain2 : Gain  Gain=2  SaturateOnIntegerOverflow=on
  Increasing index : Fcn  Expr=u(1)>0.5
  Logical Operator{,1,3..4,6..7} (6 alike) : Logic  ShowAdditionalParam=on  AllPortsSameDT=off
  Logical Operator2 : Logic  Operator=OR  ShowAdditionalParam=on  AllPortsSameDT=off  OutDataTypeMode=Specify via dialog  LogicDataType=float('double')
  Logical Operator5 : Logic  Operator=OR  ShowAdditionalParam=on  AllPortsSameDT=off  OutDataTypeMode=Specify via dialog  LogicDataType=float('double')
  Logical Operator8 : Logic  Operator=OR  ShowAdditionalParam=on  AllPortsSameDT=off  OutDataTypeMode=Specify via dialog  LogicDataType=float('double')
  Sum1 : Sum  Inputs=+++  SaturateOnIntegerOverflow=on  InputSameDT=on
  n+1 : Outport  InitialOutput=3
  wires:
  rise/fall/1 -> Falling index/1, Increasing index/1
  Gain2/1 -> Sum1/1
  Gain1/1 -> Sum1/3
  Logical Operator8/1 -> Gain1/1
  Logical Operator6/1 -> Logical Operator8/2
  Logical Operator7/1 -> Logical Operator8/1
  Gain/1 -> Sum1/2
  Logical Operator5/1 -> Gain/1
  Logical Operator3/1 -> Logical Operator5/2
  Logical Operator4/1 -> Logical Operator5/1
  Fcn2/1 -> Logical Operator7/2, Logical Operator4/2
  Logical Operator2/1 -> Gain2/1
  Sum1/1 -> n+1/1
  Logical Operator1/1 -> Logical Operator2/2
  Logical Operator/1 -> Logical Operator2/1
  Fcn3/1 -> Logical Operator3/2, Logical Operator1/2
  Falling index/1 -> Logical Operator6/1, Logical Operator4/1, Logical Operator1/1
  Fcn1/1 -> Logical Operator6/2, Logical Operator/2
  Increasing index/1 -> Logical Operator7/1, Logical Operator3/1, Logical Operator/1
  n/1 -> Fcn3/1, Fcn2/1, Fcn1/1

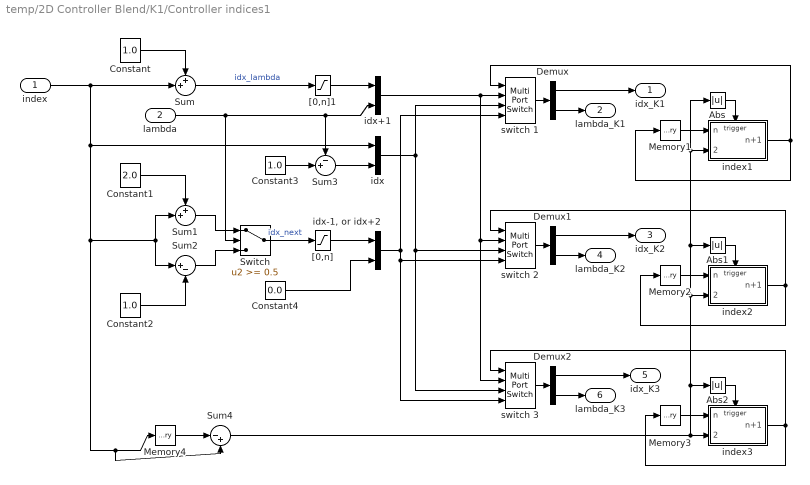
== system temp/2D Controller Blend/K1/Controller indices1 ==
  index : Inport
  lambda : Inport  Port=2
  Abs : Abs  SaturateOnIntegerOverflow=on
  Abs1 : Abs  SaturateOnIntegerOverflow=on
  Abs2 : Abs  SaturateOnIntegerOverflow=on
  Constant : Constant  Value=1.0
  Constant1 : Constant  Value=2.0
  Constant2 : Constant  Value=1.0
  Constant3 : Constant  Value=1.0
  Constant4 : Constant  Value=0.0
  Demux : Demux  Outputs=2
  Demux1 : Demux  Outputs=2
  Demux2 : Demux  Outputs=2
  Memory{1..4} (4 alike) : Memory
  Sum : Sum  Inputs=++|  SaturateOnIntegerOverflow=on  InputSameDT=on
  Sum1 : Sum  Inputs=++|  SaturateOnIntegerOverflow=on  InputSameDT=on
  Sum2 : Sum  Inputs=|+-  SaturateOnIntegerOverflow=on  InputSameDT=on
  Sum3 : Sum  Inputs=-+|  SaturateOnIntegerOverflow=on  InputSameDT=on
  Sum4 : Sum  Inputs=|-+  SaturateOnIntegerOverflow=on  InputSameDT=on
  Switch : Switch  Threshold=0.5  SaturateOnIntegerOverflow=on  InputSameDT=on
  "[0,n]" : Saturate  UpperLimit=length(breakpoints_v2)-1  LowerLimit=0
  "[0,n]1" : Saturate  UpperLimit=length(breakpoints_v2)-1  LowerLimit=0
  idx : Mux  Inputs=2
  idx+1 : Mux  Inputs=2
  "idx-1, or idx+2" : Mux  Inputs=2
  index1 : Subsystem  TreatAsAtomicUnit=on
  index2 : Subsystem  TreatAsAtomicUnit=on
  index3 : Subsystem  TreatAsAtomicUnit=on
  switch 1 : MultiPortSwitch  Inputs=3  SaturateOnIntegerOverflow=on  InputSameDT=on
  switch 2 : MultiPortSwitch  Inputs=3  SaturateOnIntegerOverflow=on  InputSameDT=on
  switch 3 : MultiPortSwitch  Inputs=3  SaturateOnIntegerOverflow=on  InputSameDT=on
  idx_K1 : Outport
  lambda_K1 : Outport  Port=2
  idx_K2 : Outport  Port=3
  lambda_K2 : Outport  Port=4
  idx_K3 : Outport  Port=5
  lambda_K3 : Outport  Port=6
  wires:
  Abs2/1 -> index3/Trigger
  Abs1/1 -> index2/Trigger
  Abs/1 -> index1/Trigger
  Sum4/1 -> Abs2/1, Abs1/1, Abs/1, index1/2(rise/fall), index2/2(rise/fall), index3/2(rise/fall)
  Memory4/1 -> Sum4/1
  "[0,n]1"/1 -> idx+1/1
  "[0,n]"/1 -> "idx-1, or idx+2"/1
  Demux2/2 -> lambda_K3/1
  Demux2/1 -> idx_K3/1
  switch 3/1 -> Demux2/1
  Demux1/2 -> lambda_K2/1
  Demux1/1 -> idx_K2/1
  switch 2/1 -> Demux1/1
  Demux/2 -> lambda_K1/1
  Demux/1 -> idx_K1/1
  switch 1/1 -> Demux/1
  "idx-1, or idx+2"/1 -> switch 3/4, switch 2/4, switch 1/4
  Constant4/1 -> "idx-1, or idx+2"/2
  Switch/1 -> "[0,n]"/1  "idx_next"
  idx/1 -> switch 3/3, switch 2/3, switch 1/3
  Constant3/1 -> Sum3/2
  Sum3/1 -> idx/2
  idx+1/1 -> switch 3/2, switch 2/2, switch 1/2
  lambda/1 -> Switch/2, Sum3/1, idx+1/2
  Sum/1 -> "[0,n]1"/1  "idx_lambda"
  index3/1(n+1) -> Memory3/1, switch 3/1
  index2/1(n+1) -> Memory2/1, switch 2/1
  Memory3/1 -> index3/1(n)
  Memory2/1 -> index2/1(n)
  index1/1(n+1) -> Memory1/1, switch 1/1
  Memory1/1 -> index1/1(n)
  Constant2/1 -> Sum2/2
  Sum2/1 -> Switch/3
  Sum1/1 -> Switch/1
  Constant1/1 -> Sum1/1
  Constant/1 -> Sum/1
  index/1 -> Sum4/2, Memory4/1, Sum2/1, Sum1/2, idx/1, Sum/2

== system temp/2D Controller Blend/K1/K1 ==
  e = refs - y : Inport  Orientation=left
  index1 : Inport  Port=2
  index2 : Inport  Port=3
  u_measured : Inport  Orientation=left  Port=4
  *A-HC : Product  Multiplication=Matrix(*)  SaturateOnIntegerOverflow=on  InputSameDT=on
  *B-HD : Product  Orientation=left  Multiplication=Matrix(*)  SaturateOnIntegerOverflow=on  InputSameDT=on
  *C : Product  Orientation=left  Multiplication=Matrix(*)  SaturateOnIntegerOverflow=on  InputSameDT=on
  *D : Product  Orientation=left  Multiplication=Matrix(*)  SaturateOnIntegerOverflow=on  InputSameDT=on
  *H : Product  Orientation=left  Multiplication=Matrix(*)  SaturateOnIntegerOverflow=on  InputSameDT=on
  A : simulink/Look-Up Tables/Direct Look-Up Table (n-D)  maskTabDims=4  explicitNumDims=3  outDims=2-D Matrix  tabIsInput=off  mxTable=A  clipFlag=Warning
  B : simulink/Look-Up Tables/Direct Look-Up Table (n-D)  maskTabDims=4  explicitNumDims=3  outDims=2-D Matrix  tabIsInput=off  mxTable=B  clipFlag=Warning
  C : simulink/Look-Up Tables/Direct Look-Up Table (n-D)  maskTabDims=4  explicitNumDims=3  outDims=2-D Matrix  tabIsInput=off  mxTable=C  clipFlag=Warning
  D : simulink/Look-Up Tables/Direct Look-Up Table (n-D)  maskTabDims=4  explicitNumDims=3  outDims=2-D Matrix  tabIsInput=off  mxTable=D  clipFlag=Warning
  Estimated state : Integrator  Orientation=left  InitialCondition=x_initial
  H : simulink/Look-Up Tables/Direct Look-Up Table (n-D)  maskTabDims=4  explicitNumDims=3  outDims=2-D Matrix  tabIsInput=off  mxTable=H  clipFlag=Warning
  H*C : Product  Multiplication=Matrix(*)  SaturateOnIntegerOverflow=on  InputSameDT=on
  H*D : Product  Multiplication=Matrix(*)  SaturateOnIntegerOverflow=on  InputSameDT=on
  Sum : Sum  Orientation=left  Inputs=+++  SaturateOnIntegerOverflow=on  InputSameDT=on
  Sum1 : Sum  Inputs=-+|  SaturateOnIntegerOverflow=on  InputSameDT=on
  Sum2 : Sum  Orientation=left  Inputs=|++  SaturateOnIntegerOverflow=on  InputSameDT=on
  Sum3 : Sum  Inputs=-+|  SaturateOnIntegerOverflow=on  InputSameDT=on
  u_demand : Outport  Orientation=left
  wires:
  D/1 -> *D/1, H*D/2
  Sum2/1 -> u_demand/1
  *D/1 -> Sum2/2
  *C/1 -> Sum2/1
  index1/1 -> C/1, A/1, D/1, B/1, H/1
  e = refs - y/1 -> *D/2, *B-HD/2
  C/1 -> *C/1, H*C/2
  Estimated state/1 -> *A-HC/2, *C/2
  Sum/1 -> Estimated state/1
  *A-HC/1 -> Sum/3
  *B-HD/1 -> Sum/2
  *H/1 -> Sum/1
  u_measured/1 -> *H/2
  H/1 -> *H/1, H*D/1, H*C/1
  H*D/1 -> Sum1/1
  B/1 -> Sum1/2
  Sum1/1 -> *B-HD/1
  A/1 -> Sum3/2
  Sum3/1 -> *A-HC/1
  H*C/1 -> Sum3/1
  index2/1 -> H/2, B/2, D/2, C/2, A/2

== system temp/2D Controller Blend/K1/Controller indices1/index1 ==
  n : Inport
  rise/fall : Inport  Port=2
  Trigger : TriggerPort
  Falling index : Fcn  Expr=u(1)<-0.5
  Fcn1 : Fcn  Expr=u(1)==1
  Fcn2 : Fcn  Expr=u(1)==2
  Fcn3 : Fcn  Expr=u(1)==3
  Gain : Gain  SaturateOnIntegerOverflow=on
  Gain1 : Gain  Gain=3  SaturateOnIntegerOverflow=on
  Gain2 : Gain  Gain=2  SaturateOnIntegerOverflow=on
  Increasing index : Fcn  Expr=u(1)>0.5
  Logical Operator{,1,3..4,6..7} (6 alike) : Logic  ShowAdditionalParam=on  AllPortsSameDT=off
  Logical Operator2 : Logic  Operator=OR  ShowAdditionalParam=on  AllPortsSameDT=off  OutDataTypeMode=Specify via dialog  LogicDataType=float('double')
  Logical Operator5 : Logic  Operator=OR  ShowAdditionalParam=on  AllPortsSameDT=off  OutDataTypeMode=Specify via dialog  LogicDataType=float('double')
  Logical Operator8 : Logic  Operator=OR  ShowAdditionalParam=on  AllPortsSameDT=off  OutDataTypeMode=Specify via dialog  LogicDataType=float('double')
  Sum1 : Sum  Inputs=+++  SaturateOnIntegerOverflow=on  InputSameDT=on
  n+1 : Outport  InitialOutput=1
  wires:
  rise/fall/1 -> Falling index/1, Increasing index/1
  Gain2/1 -> Sum1/1
  Gain1/1 -> Sum1/3
  Logical Operator8/1 -> Gain1/1
  Logical Operator6/1 -> Logical Operator8/2
  Logical Operator7/1 -> Logical Operator8/1
  Gain/1 -> Sum1/2
  Logical Operator5/1 -> Gain/1
  Logical Operator3/1 -> Logical Operator5/2
  Logical Operator4/1 -> Logical Operator5/1
  Fcn2/1 -> Logical Operator7/2, Logical Operator4/2
  Logical Operator2/1 -> Gain2/1
  Sum1/1 -> n+1/1
  Logical Operator1/1 -> Logical Operator2/2
  Logical Operator/1 -> Logical Operator2/1
  Fcn3/1 -> Logical Operator3/2, Logical Operator1/2
  Falling index/1 -> Logical Operator6/1, Logical Operator4/1, Logical Operator1/1
  Fcn1/1 -> Logical Operator6/2, Logical Operator/2
  Increasing index/1 -> Logical Operator7/1, Logical Operator3/1, Logical Operator/1
  n/1 -> Fcn3/1, Fcn2/1, Fcn1/1

== system temp/2D Controller Blend/K1/Controller indices1/index2 ==
  n : Inport
  rise/fall : Inport  Port=2
  Trigger : TriggerPort
  Falling index : Fcn  Expr=u(1)<-0.5
  Fcn1 : Fcn  Expr=u(1)==1
  Fcn2 : Fcn  Expr=u(1)==2
  Fcn3 : Fcn  Expr=u(1)==3
  Gain : Gain  SaturateOnIntegerOverflow=on
  Gain1 : Gain  Gain=3  SaturateOnIntegerOverflow=on
  Gain2 : Gain  Gain=2  SaturateOnIntegerOverflow=on
  Increasing index : Fcn  Expr=u(1)>0.5
  Logical Operator{,1,3..4,6..7} (6 alike) : Logic  ShowAdditionalParam=on  AllPortsSameDT=off
  Logical Operator2 : Logic  Operator=OR  ShowAdditionalParam=on  AllPortsSameDT=off  OutDataTypeMode=Specify via dialog  LogicDataType=float('double')
  Logical Operator5 : Logic  Operator=OR  ShowAdditionalParam=on  AllPortsSameDT=off  OutDataTypeMode=Specify via dialog  LogicDataType=float('double')
  Logical Operator8 : Logic  Operator=OR  ShowAdditionalParam=on  AllPortsSameDT=off  OutDataTypeMode=Specify via dialog  LogicDataType=float('double')
  Sum1 : Sum  Inputs=+++  SaturateOnIntegerOverflow=on  InputSameDT=on
  n+1 : Outport  InitialOutput=2
  wires:
  n/1 -> Fcn1/1, Fcn2/1, Fcn3/1
  Increasing index/1 -> Logical Operator/1, Logical Operator3/1, Logical Operator7/1
  Fcn1/1 -> Logical Operator/2, Logical Operator6/2
  Falling index/1 -> Logical Operator1/1, Logical Operator4/1, Logical Operator6/1
  Fcn3/1 -> Logical Operator1/2, Logical Operator3/2
  Logical Operator/1 -> Logical Operator2/1
  Logical Operator1/1 -> Logical Operator2/2
  Sum1/1 -> n+1/1
  Logical Operator2/1 -> Gain2/1
  Fcn2/1 -> Logical Operator4/2, Logical Operator7/2
  Logical Operator4/1 -> Logical Operator5/1
  Logical Operator3/1 -> Logical Operator5/2
  Logical Operator5/1 -> Gain/1
  Gain/1 -> Sum1/2
  Logical Operator7/1 -> Logical Operator8/1
  Logical Operator6/1 -> Logical Operator8/2
  Logical Operator8/1 -> Gain1/1
  Gain1/1 -> Sum1/3
  Gain2/1 -> Sum1/1
  rise/fall/1 -> Increasing index/1, Falling index/1

== system temp/2D Controller Blend/K1/Controller indices1/index3 ==
  n : Inport
  rise/fall : Inport  Port=2
  Trigger : TriggerPort
  Falling index : Fcn  Expr=u(1)<-0.5
  Fcn1 : Fcn  Expr=u(1)==1
  Fcn2 : Fcn  Expr=u(1)==2
  Fcn3 : Fcn  Expr=u(1)==3
  Gain : Gain  SaturateOnIntegerOverflow=on
  Gain1 : Gain  Gain=3  SaturateOnIntegerOverflow=on
  Gain2 : Gain  Gain=2  SaturateOnIntegerOverflow=on
  Increasing index : Fcn  Expr=u(1)>0.5
  Logical Operator{,1,3..4,6..7} (6 alike) : Logic  ShowAdditionalParam=on  AllPortsSameDT=off
  Logical Operator2 : Logic  Operator=OR  ShowAdditionalParam=on  AllPortsSameDT=off  OutDataTypeMode=Specify via dialog  LogicDataType=float('double')
  Logical Operator5 : Logic  Operator=OR  ShowAdditionalParam=on  AllPortsSameDT=off  OutDataTypeMode=Specify via dialog  LogicDataType=float('double')
  Logical Operator8 : Logic  Operator=OR  ShowAdditionalParam=on  AllPortsSameDT=off  OutDataTypeMode=Specify via dialog  LogicDataType=float('double')
  Sum1 : Sum  Inputs=+++  SaturateOnIntegerOverflow=on  InputSameDT=on
  n+1 : Outport  InitialOutput=3
  wires:
  rise/fall/1 -> Falling index/1, Increasing index/1
  Gain2/1 -> Sum1/1
  Gain1/1 -> Sum1/3
  Logical Operator8/1 -> Gain1/1
  Logical Operator6/1 -> Logical Operator8/2
  Logical Operator7/1 -> Logical Operator8/1
  Gain/1 -> Sum1/2
  Logical Operator5/1 -> Gain/1
  Logical Operator3/1 -> Logical Operator5/2
  Logical Operator4/1 -> Logical Operator5/1
  Fcn2/1 -> Logical Operator7/2, Logical Operator4/2
  Logical Operator2/1 -> Gain2/1
  Sum1/1 -> n+1/1
  Logical Operator1/1 -> Logical Operator2/2
  Logical Operator/1 -> Logical Operator2/1
  Fcn3/1 -> Logical Operator3/2, Logical Operator1/2
  Falling index/1 -> Logical Operator6/1, Logical Operator4/1, Logical Operator1/1
  Fcn1/1 -> Logical Operator6/2, Logical Operator/2
  Increasing index/1 -> Logical Operator7/1, Logical Operator3/1, Logical Operator/1
  n/1 -> Fcn3/1, Fcn2/1, Fcn1/1
